simulink model "rtwdemo_switcheml"  (Simulink 7.1)
settings: Solver=FixedStepDiscrete  StartTime=0.0  StopTime=10.0  FixedStep=.01  RelTol=1e-3
settings Model: Creator=ajayaram  LastModifiedBy=ajayaram
settings SolverCC: AutoInsertRateTranBlk=on
settings DataIOCC: SaveOutput=off  SaveTime=off
settings OptimizationCC: InlineParams=on  InlineInvariantSignals=on  EnforceIntegerDowncast=off  StateBitsets=on  DataBitsets=on  UseTempVars=on  OptimizeModelRefInitCode=on  LifeSpan=1
settings DebuggingCC: SaveWithParameterizedLinksMsg=none
settings RTWCC: SystemTargetFile=ert.tlc  GenCodeOnly=on  GenerateMakefile=off  TemplateMakefile=ert_default_tmf  Description=Real-Time Workshop Embedded Coder (no auto configuration)  GenerateReport=on  RTWVerbose=off  ProcessScript=ert_make_rtw_hook  IncludeHyperlinkInReport=on  LaunchReport=on
settings CodeAppCC: GenerateComments=off  IgnoreCustomStorageClasses=off  CustomSymbolStrGlobalVar=rt$N$M  CustomSymbolStrType=$N$M  CustomSymbolStrFcn=$N$M$F  CustomSymbolStrMacro=$N$M  SimulinkBlockComments=off
settings ERTTargetCC: GenerateSampleERTMain=on  SuppressErrorStatus=on  SupportAbsoluteTime=off  SupportNonFinite=off  SupportComplex=off  InlinedParameterPlacement=NonHierarchical  RootIOFormat=Structure reference  ERTCustomFileTemplate=example_file_process.tlc

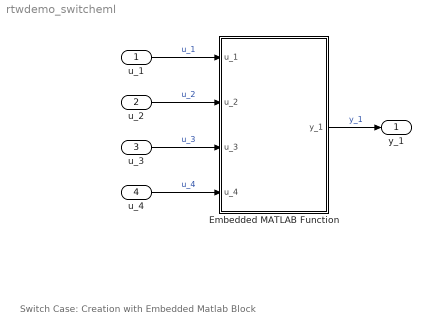
== system rtwdemo_switcheml ==
  note: Switch Case: Creation with
      | Embedded Matlab Block
  u_1 : Inport  DataType=uint32  OutDataType=sfix(16)  OutScaling=2^0  OutDataTypeStr=uint32
  u_2 : Inport  Port=2  OutDataType=sfix(16)  OutScaling=2^0
  u_3 : Inport  Port=3  OutDataType=sfix(16)  OutScaling=2^0
  u_4 : Inport  Port=4  OutDataType=sfix(16)  OutScaling=2^0
  Embedded MATLAB Function : Stateflow chart
  y_1 : Outport  OutDataType=sfix(16)  OutScaling=2^0
  wires:
  u_1/1 -> Embedded MATLAB Function/1(u_1)  "u_1"
  u_2/1 -> Embedded MATLAB Function/2(u_2)  "u_2"
  u_3/1 -> Embedded MATLAB Function/3(u_3)  "u_3"
  u_4/1 -> Embedded MATLAB Function/4(u_4)  "u_4"
  Embedded MATLAB Function/1(y_1) -> y_1/1  "y_1"

== matlab function Embedded MATLAB Function ==
  data: u_1 input double; u_2 input double; u_3 input double; u_4 input double; y_1 output double
function y_1 = fcn(u_1,u_2,u_3,u_4)

switch u_1
    case 2
        y_1 = u_2;
    case 3
        y_1 = u_3;
    otherwise
        y_1 = u_4;
end
